simulink model "IntegratedSim2"  (R2018a)
settings: Solver=ode45  StartTime=0.0  StopTime=25  RelTol=1e-7
undefined symbols (not defined in the file or in its folder): Hsys0, qBody0, vp
libraries: vrlib x4, aerolibutil x2, dspmtrx3 x1
settings Model: Creator=henry  LastModifiedBy=henry
settings SolverCC: ConsecutiveZCsStepRelTol=10*128*1  ZeroCrossControl=EnableAll  ZeroCrossAlgorithm=Adaptive

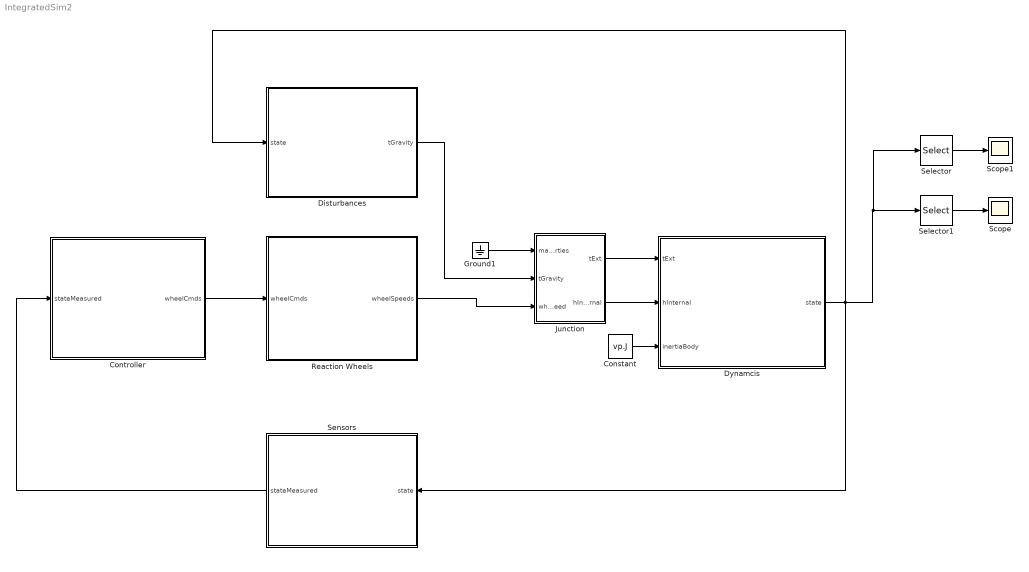
== system IntegratedSim2 ==
  Constant : Constant  Value=vp.J
  Controller : Subsystem
  Disturbances : Subsystem
  Dynamcis : Subsystem
  Ground1 : Ground
  Junction : Subsystem
  Reaction Wheels : Subsystem
  Scope : Scope
  Scope1 : Scope
  Selector : Selector  InputPortWidth=7  IndexOptions=Index vector (dialog)  Indices=[1:4]  OutputSizes=1
  Selector1 : Selector  InputPortWidth=7  IndexOptions=Index vector (dialog)  Indices=[5:7]  OutputSizes=1
  Sensors : Subsystem
  wires:
  Disturbances/1(tGravity) -> Junction/2(tGravity)
  Ground1/1 -> Junction/1(massProperties)
  Junction/1(tExt) -> Dynamcis/1(tExt)
  Controller/1(wheelCmds) -> Reaction Wheels/1(wheelCmds)
  Reaction Wheels/1(wheelSpeeds) -> Junction/3(wheelSpeed)
  Sensors/1(stateMeasured) -> Controller/1(stateMeasured)
  Constant/1 -> Dynamcis/3(inertiaBody)
  Junction/2(hInternal) -> Dynamcis/2(hInternal)
  Dynamcis/1(state) -> Selector/1, Selector1/1, Disturbances/1("state "), Sensors/1(state)
  Selector1/1 -> Scope/1
  Selector/1 -> Scope1/1

== system IntegratedSim2/Controller ==
  stateMeasured : Inport
  wheelCmds : Outport
  wires:
  stateMeasured/1 -> wheelCmds/1

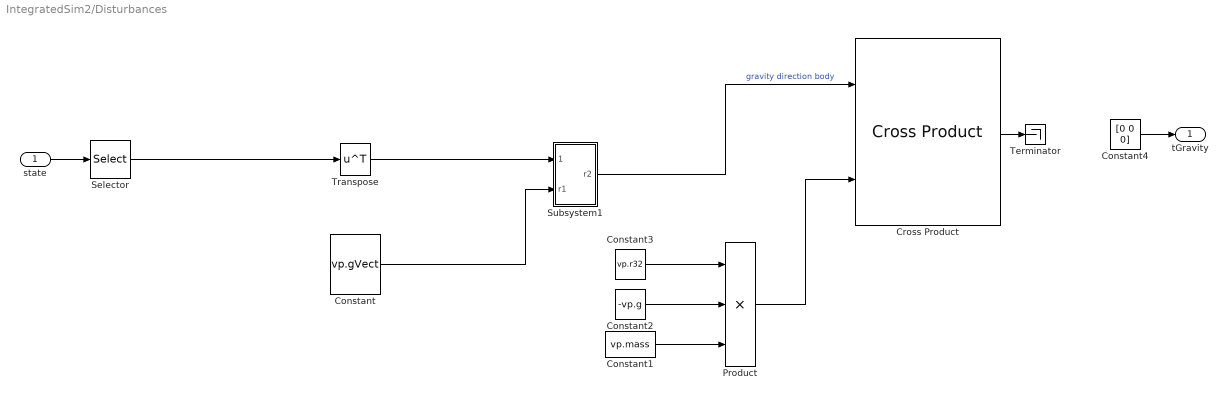
== system IntegratedSim2/Disturbances ==
  "state " : Inport
  Constant : Constant  Value=vp.gVect
  Constant1 : Constant  Value=vp.mass
  Constant2 : Constant  Value=-vp.g
  Constant3 : Constant  Value=vp.r32
  Constant4 : Constant  Value=[0 0 0]
  Cross Product : vrlib/Utilities/Cross Product
      settings: SourceProductBaseCode=VR
  Product : Product  Inputs=3
  Selector : Selector  InputPortWidth=7  IndexOptions=Index vector (dialog)  Indices=[1:4]  OutputSizes=1
  Subsystem1 : Subsystem  mask(Quaternion Transformation){}
      mask help: This blocks transforms the vector r1 from frame a to frame b.
  Terminator : Terminator
  Transpose : Math  Operator=transpose  SaturateOnIntegerOverflow=on
  tGravity : Outport
  wires:
  Constant/1 -> Subsystem1/2(r1)
  Constant1/1 -> Product/3
  Constant2/1 -> Product/2
  Constant3/1 -> Product/1
  Transpose/1 -> Subsystem1/1(qa2b)
  "state "/1 -> Selector/1
  Selector/1 -> Transpose/1
  Product/1 -> Cross Product/2
  Subsystem1/1(r2) -> Cross Product/1  "gravity direction body"
  Constant4/1 -> tGravity/1
  Cross Product/1 -> Terminator/1

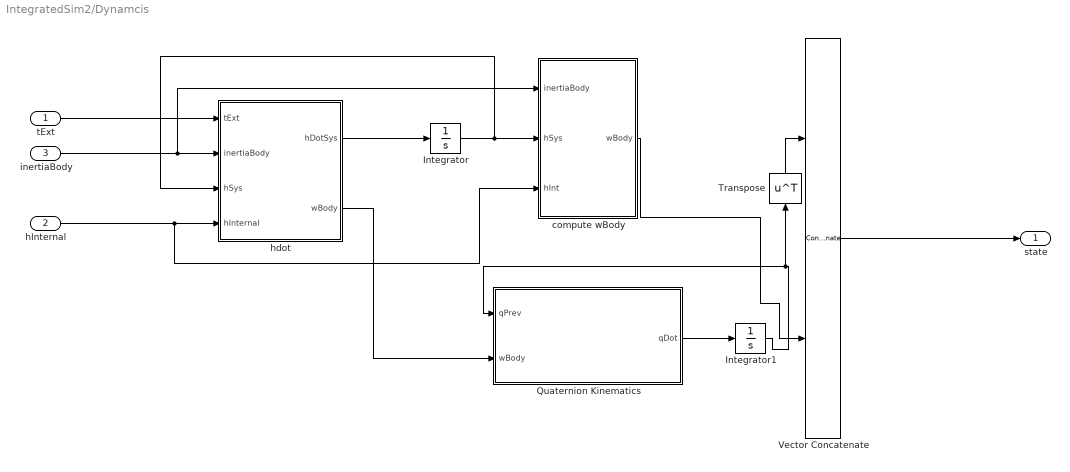
== system IntegratedSim2/Dynamcis ==
  tExt : Inport
  hInternal : Inport  Port=2
  inertiaBody : Inport  Port=3
  Integrator : Integrator  InitialCondition=Hsys0
  Integrator1 : Integrator  InitialCondition=qBody0
  Quaternion Kinematics : Subsystem
  Transpose : Math  Operator=transpose  SaturateOnIntegerOverflow=on
  Vector Concatenate : Concatenate
  compute wBody : Subsystem
  hdot : Subsystem
  state : Outport
  wires:
  hInternal/1 -> compute wBody/3(hInt), hdot/4(hInternal)
  inertiaBody/1 -> compute wBody/1(inertiaBody), hdot/2(inertiaBody)
  tExt/1 -> hdot/1(tExt)
  hdot/1(hDotSys) -> Integrator/1
  Quaternion Kinematics/1(qDot) -> Integrator1/1
  hdot/2(wBody) -> Quaternion Kinematics/2(wBody)
  Integrator/1 -> hdot/3(hSys), compute wBody/2(hSys)
  Integrator1/1 -> Transpose/1, Quaternion Kinematics/1(qPrev)
  Vector Concatenate/1 -> state/1
  compute wBody/1(wBody) -> Vector Concatenate/2
  Transpose/1 -> Vector Concatenate/1

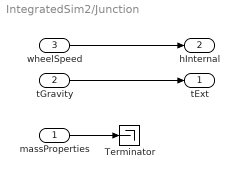
== system IntegratedSim2/Junction ==
  massProperties : Inport
  tGravity : Inport  Port=2
  wheelSpeed : Inport  Port=3
  Terminator : Terminator
  tExt : Outport
  hInternal : Outport  Port=2
  wires:
  wheelSpeed/1 -> hInternal/1
  tGravity/1 -> tExt/1
  massProperties/1 -> Terminator/1

== system IntegratedSim2/Reaction Wheels ==
  wheelCmds : Inport
  Constant : Constant  Value=[0 0 0]
  Terminator : Terminator
  wheelSpeeds : Outport
  wires:
  wheelCmds/1 -> Terminator/1
  Constant/1 -> wheelSpeeds/1

== system IntegratedSim2/Sensors ==
  state : Inport
  stateMeasured : Outport
  wires:
  state/1 -> stateMeasured/1

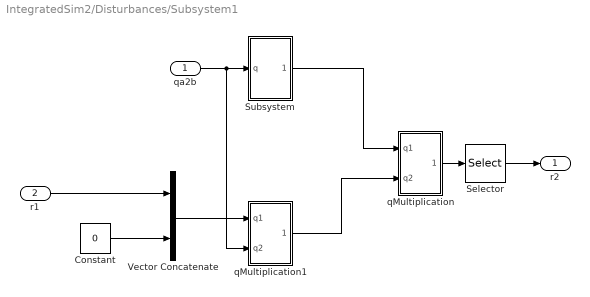
== system IntegratedSim2/Disturbances/Subsystem1 ==
  qa2b : Inport
  r1 : Inport  Port=2
  Constant : Constant  Value=0
  Selector : Selector  InputPortWidth=4  IndexOptions=Index vector (dialog)  Indices=[1:3]  OutputSizes=1
  Subsystem : Subsystem  mask(Quaternion Conjugate){}
      mask help: This block takes the conjugate of the input quaternion
  Vector Concatenate : Concatenate
  qMultiplication : Subsystem  mask(Quaternion Multiplication){}
      mask help: This block performs the quaternion multiplication given two input quaternions.
  qMultiplication1 : Subsystem  mask(Quaternion Multiplication){}
      mask help: This block performs the quaternion multiplication given two input quaternions.
  r2 : Outport
  wires:
  Selector/1 -> r2/1
  qMultiplication/1(q12) -> Selector/1
  qMultiplication1/1(q12) -> qMultiplication/2(q2)
  Vector Concatenate/1 -> qMultiplication1/1(q1)
  Constant/1 -> Vector Concatenate/2
  Subsystem/1(qConj) -> qMultiplication/1(q1)
  qa2b/1 -> Subsystem/1(q), qMultiplication1/2(q2)
  r1/1 -> Vector Concatenate/1

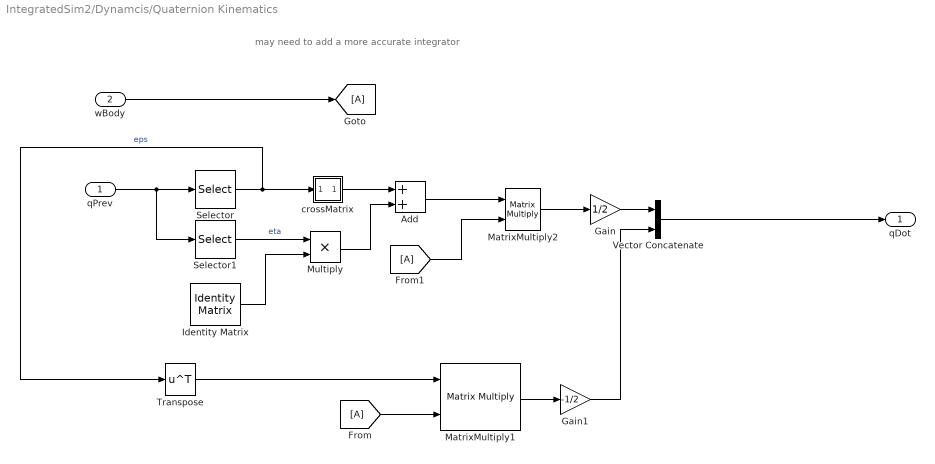
== system IntegratedSim2/Dynamcis/Quaternion Kinematics ==
  note: may need to add a more accurate integrator
  qPrev : Inport
  wBody : Inport  Port=2
  Add : Sum
  Gain : Gain  Gain=1/2
  Gain1 : Gain  Gain=-1/2
  Identity Matrix : dspmtrx3/Identity Matrix  Inherit=off  N=3  Ts=1  dataType=double  isSigned=on  wordLen=16  udDataType=sfix(16)  fracBitsMode=Best precision  numFracBits=15  OutDataTypeStr=double  LastOutDataTypeStr=double
      settings: SourceProductName=DSP System Toolbox
  MatrixMultiply1 : Product  Multiplication=Matrix(*)
  MatrixMultiply2 : Product  Multiplication=Matrix(*)
  Multiply : Product
  Selector : Selector  InputPortWidth=4  IndexOptions=Index vector (dialog)  Indices=[1:3]  OutputSizes=1
  Selector1 : Selector  InputPortWidth=4  IndexOptions=Index vector (dialog)  Indices=4  OutputSizes=1
  Transpose : Math  Operator=transpose  SaturateOnIntegerOverflow=on
  Vector Concatenate : Concatenate
  "crossMatrix " : Subsystem  mask(Cross Matrix){}
      mask help: This block takes in a 3x1 vector and outputs it's corresponding 3x3 cross product matrix
  qDot : Outport
  wires:
  qPrev/1 -> Selector1/1, Selector/1
  Selector/1 -> Transpose/1, "crossMatrix "/1(a)  "eps"
  Selector1/1 -> Multiply/1  "eta"
  Identity Matrix/1 -> Multiply/2
  "crossMatrix "/1(aX) -> Add/1
  Multiply/1 -> Add/2
  Add/1 -> MatrixMultiply2/1
  MatrixMultiply2/1 -> Gain/1
  Gain/1 -> Vector Concatenate/1
  MatrixMultiply1/1 -> Gain1/1
  Gain1/1 -> Vector Concatenate/2
  [A] -> MatrixMultiply1/2
  [A] -> MatrixMultiply2/2
  wBody/1 -> [A]
  Vector Concatenate/1 -> qDot/1
  Transpose/1 -> MatrixMultiply1/1

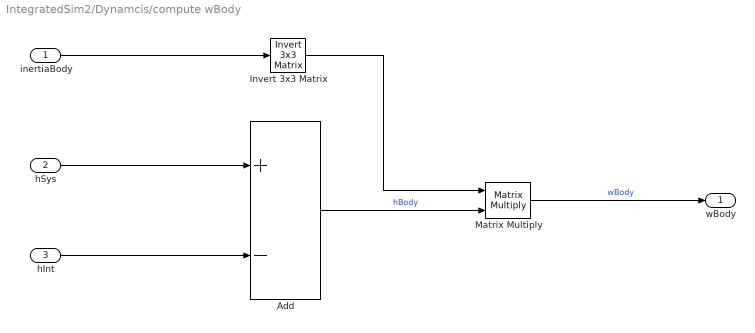
== system IntegratedSim2/Dynamcis/compute wBody ==
  inertiaBody : Inport
  hSys : Inport  Port=2
  hInt : Inport  Port=3
  Add : Sum  Inputs=+-
  Invert 3x3 Matrix : aerolibutil/Invert  3x3 Matrix
  Matrix Multiply : Product  Multiplication=Matrix(*)
  wBody : Outport
  wires:
  inertiaBody/1 -> Invert 3x3 Matrix/1
  hSys/1 -> Add/1
  Matrix Multiply/1 -> wBody/1  "wBody"
  Invert 3x3 Matrix/1 -> Matrix Multiply/1
  hInt/1 -> Add/2
  Add/1 -> Matrix Multiply/2  "hBody"

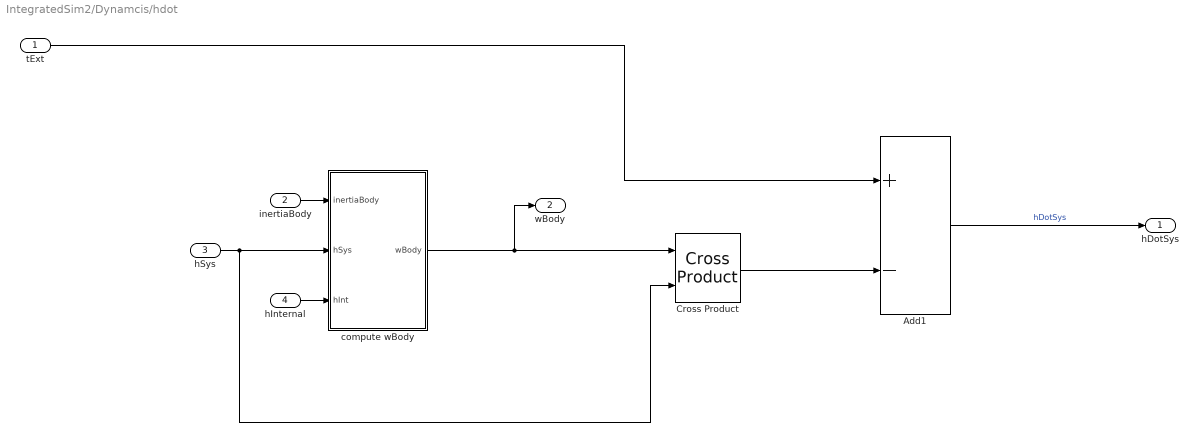
== system IntegratedSim2/Dynamcis/hdot ==
  tExt : Inport
  inertiaBody : Inport  Port=2
  hSys : Inport  Port=3
  hInternal : Inport  Port=4
  Add1 : Sum  Inputs=+-
  Cross Product : vrlib/Utilities/Cross Product
      settings: SourceProductBaseCode=VR
  compute wBody : Subsystem
  hDotSys : Outport
  wBody : Outport  Port=2
  wires:
  Add1/1 -> hDotSys/1  "hDotSys"
  tExt/1 -> Add1/1
  Cross Product/1 -> Add1/2
  inertiaBody/1 -> compute wBody/1(inertiaBody)
  hInternal/1 -> compute wBody/3(hInt)
  compute wBody/1(wBody) -> wBody/1, Cross Product/1
  hSys/1 -> Cross Product/2, compute wBody/2(hSys)

== system IntegratedSim2/Disturbances/Subsystem1/Subsystem ==
  q : Inport
  Gain : Gain  Gain=-1
  Selector : Selector  InputPortWidth=4  IndexOptions=Index vector (dialog)  Indices=[1:3]  OutputSizes=1
  Selector1 : Selector  InputPortWidth=4  IndexOptions=Index vector (dialog)  Indices=4  OutputSizes=1
  Vector Concatenate : Concatenate
  qConj : Outport
  wires:
  Vector Concatenate/1 -> qConj/1
  Gain/1 -> Vector Concatenate/1
  Selector1/1 -> Vector Concatenate/2
  q/1 -> Selector1/1, Selector/1
  Selector/1 -> Gain/1

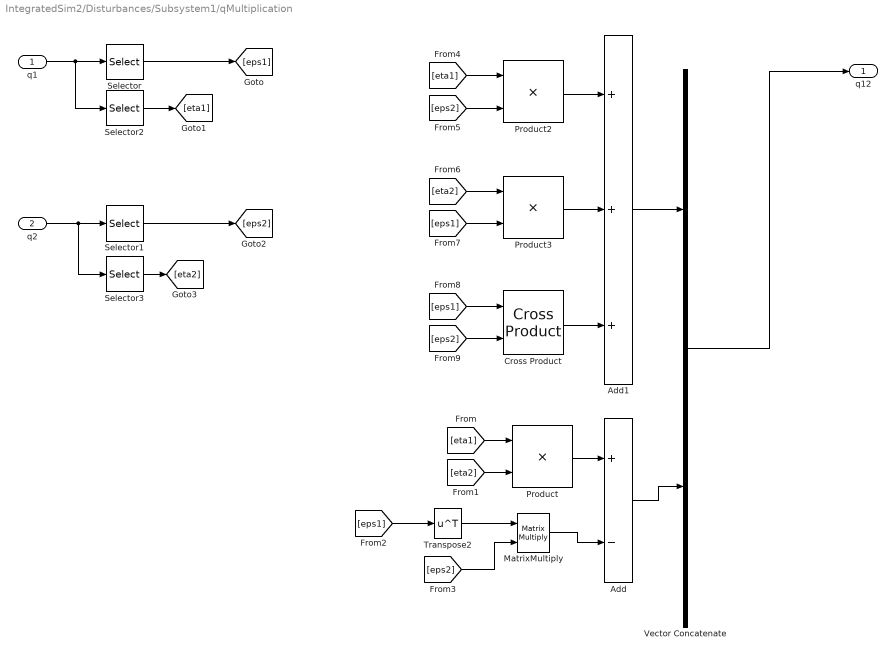
== system IntegratedSim2/Disturbances/Subsystem1/qMultiplication ==
  q1 : Inport
  q2 : Inport  Port=2
  Add : Sum  Inputs=+-
  Add1 : Sum  Inputs=+++
  Cross Product : vrlib/Utilities/Cross Product
      settings: SourceProductBaseCode=VR
  MatrixMultiply : Product  Multiplication=Matrix(*)
  Product : Product
  Product2 : Product
  Product3 : Product
  Selector : Selector  InputPortWidth=4  IndexOptions=Index vector (dialog)  Indices=[1:3]  OutputSizes=1
  Selector1 : Selector  InputPortWidth=4  IndexOptions=Index vector (dialog)  Indices=[1:3]  OutputSizes=1
  Selector2 : Selector  InputPortWidth=4  IndexOptions=Index vector (dialog)  Indices=4  OutputSizes=1
  Selector3 : Selector  InputPortWidth=4  IndexOptions=Index vector (dialog)  Indices=4  OutputSizes=1
  Transpose2 : Math  Operator=transpose  SaturateOnIntegerOverflow=on
  Vector Concatenate : Concatenate
  q12 : Outport
  wires:
  Selector3/1 -> [eta2]
  Product2/1 -> Add1/1
  Product/1 -> Add/1
  [eta1] -> Product2/1
  [eta2] -> Product/2
  Product3/1 -> Add1/2
  q1/1 -> Selector2/1, Selector/1
  Transpose2/1 -> MatrixMultiply/1
  Selector2/1 -> [eta1]
  Selector1/1 -> [eps2]
  Cross Product/1 -> Add1/3
  [eps1] -> Transpose2/1
  q2/1 -> Selector3/1, Selector1/1
  [eta2] -> Product3/1
  [eta1] -> Product/1
  Vector Concatenate/1 -> q12/1
  [eps2] -> Product2/2
  [eps1] -> Product3/2
  Selector/1 -> [eps1]
  [eps2] -> Cross Product/2
  MatrixMultiply/1 -> Add/2
  [eps1] -> Cross Product/1
  [eps2] -> MatrixMultiply/2
  Add1/1 -> Vector Concatenate/1
  Add/1 -> Vector Concatenate/2

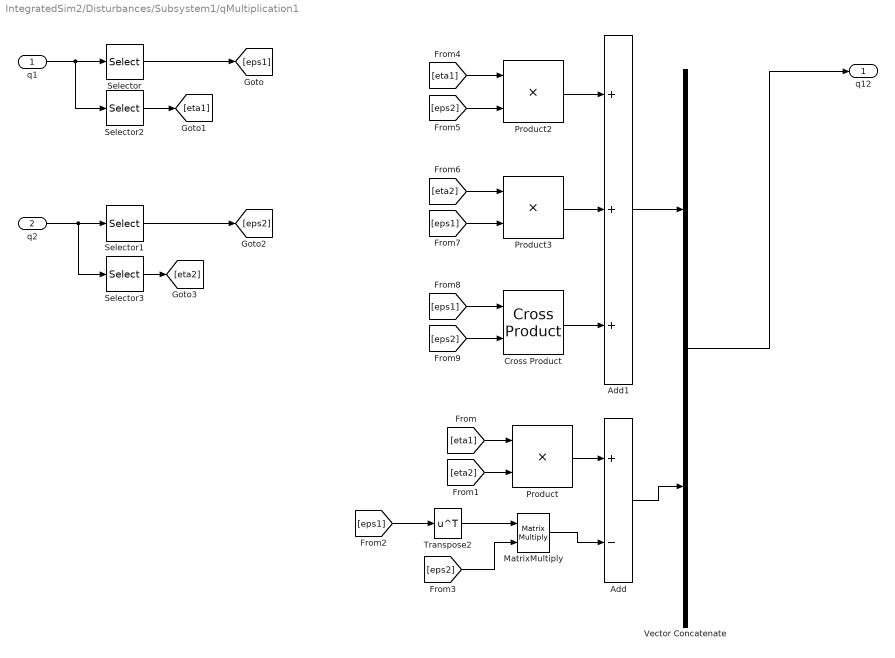
== system IntegratedSim2/Disturbances/Subsystem1/qMultiplication1 ==
  q1 : Inport
  q2 : Inport  Port=2
  Add : Sum  Inputs=+-
  Add1 : Sum  Inputs=+++
  Cross Product : vrlib/Utilities/Cross Product
      settings: SourceProductBaseCode=VR
  MatrixMultiply : Product  Multiplication=Matrix(*)
  Product : Product
  Product2 : Product
  Product3 : Product
  Selector : Selector  InputPortWidth=4  IndexOptions=Index vector (dialog)  Indices=[1:3]  OutputSizes=1
  Selector1 : Selector  InputPortWidth=4  IndexOptions=Index vector (dialog)  Indices=[1:3]  OutputSizes=1
  Selector2 : Selector  InputPortWidth=4  IndexOptions=Index vector (dialog)  Indices=4  OutputSizes=1
  Selector3 : Selector  InputPortWidth=4  IndexOptions=Index vector (dialog)  Indices=4  OutputSizes=1
  Transpose2 : Math  Operator=transpose  SaturateOnIntegerOverflow=on
  Vector Concatenate : Concatenate
  q12 : Outport
  wires:
  Add/1 -> Vector Concatenate/2
  Add1/1 -> Vector Concatenate/1
  [eps2] -> MatrixMultiply/2
  [eps1] -> Cross Product/1
  MatrixMultiply/1 -> Add/2
  [eps2] -> Cross Product/2
  Selector/1 -> [eps1]
  [eps1] -> Product3/2
  [eps2] -> Product2/2
  Vector Concatenate/1 -> q12/1
  [eta1] -> Product/1
  [eta2] -> Product3/1
  q2/1 -> Selector1/1, Selector3/1
  [eps1] -> Transpose2/1
  Cross Product/1 -> Add1/3
  Selector1/1 -> [eps2]
  Selector2/1 -> [eta1]
  Transpose2/1 -> MatrixMultiply/1
  q1/1 -> Selector/1, Selector2/1
  Product3/1 -> Add1/2
  [eta2] -> Product/2
  [eta1] -> Product2/1
  Product/1 -> Add/1
  Product2/1 -> Add1/1
  Selector3/1 -> [eta2]

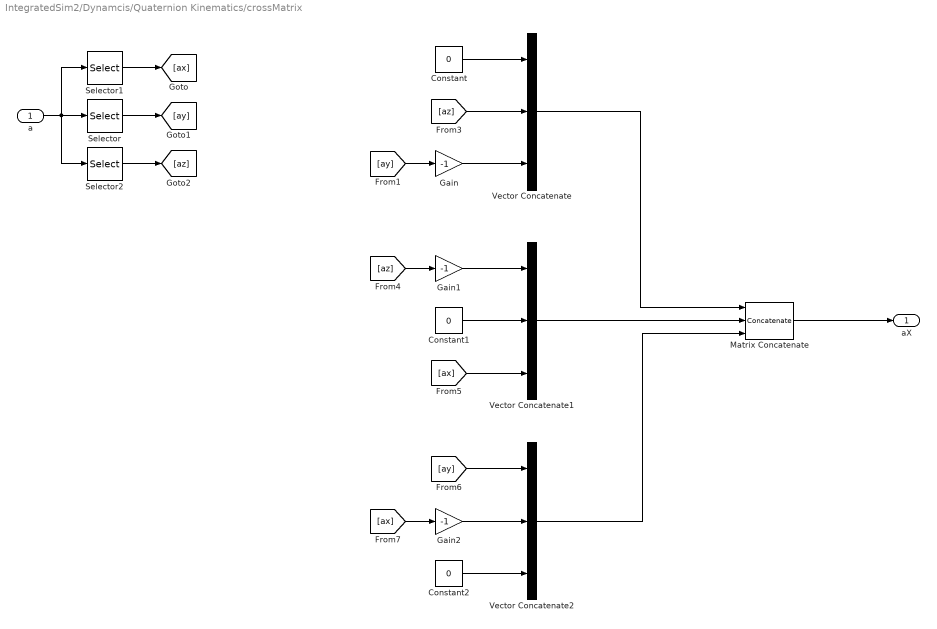
== system IntegratedSim2/Dynamcis/Quaternion Kinematics/crossMatrix  ==
  a : Inport
  Constant : Constant  Value=0
  Constant1 : Constant  Value=0
  Constant2 : Constant  Value=0
  Gain : Gain  Gain=-1
  Gain1 : Gain  Gain=-1
  Gain2 : Gain  Gain=-1
  Matrix Concatenate : Concatenate  NumInputs=3  Mode=Multidimensional array  ConcatenateDimension=2
  Selector : Selector  InputPortWidth=3  IndexOptions=Index vector (dialog)  Indices=2  OutputSizes=1
  Selector1 : Selector  InputPortWidth=3  IndexOptions=Index vector (dialog)  Indices=1  OutputSizes=1
  Selector2 : Selector  InputPortWidth=3  IndexOptions=Index vector (dialog)  Indices=3  OutputSizes=1
  Vector Concatenate : Concatenate  NumInputs=3
  Vector Concatenate1 : Concatenate  NumInputs=3
  Vector Concatenate2 : Concatenate  NumInputs=3
  aX : Outport
  wires:
  [ay] -> Gain/1
  [az] -> Gain1/1
  Gain2/1 -> Vector Concatenate2/2
  Constant1/1 -> Vector Concatenate1/2
  [ax] -> Vector Concatenate1/3
  [ay] -> Vector Concatenate2/1
  Vector Concatenate1/1 -> Matrix Concatenate/2
  Matrix Concatenate/1 -> aX/1
  Constant2/1 -> Vector Concatenate2/3
  [ax] -> Gain2/1
  Vector Concatenate2/1 -> Matrix Concatenate/3
  Gain/1 -> Vector Concatenate/3
  Vector Concatenate/1 -> Matrix Concatenate/1
  Selector1/1 -> [ax]
  Selector2/1 -> [az]
  [az] -> Vector Concatenate/2
  Gain1/1 -> Vector Concatenate1/1
  Constant/1 -> Vector Concatenate/1
  a/1 -> Selector/1, Selector1/1, Selector2/1
  Selector/1 -> [ay]

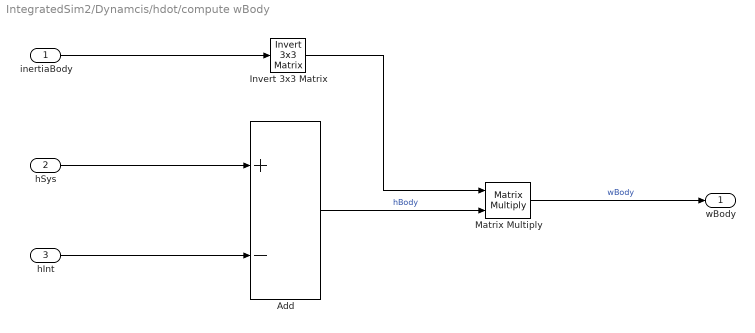
== system IntegratedSim2/Dynamcis/hdot/compute wBody ==
  inertiaBody : Inport
  hSys : Inport  Port=2
  hInt : Inport  Port=3
  Add : Sum  Inputs=+-
  Invert 3x3 Matrix : aerolibutil/Invert  3x3 Matrix
  Matrix Multiply : Product  Multiplication=Matrix(*)
  wBody : Outport
  wires:
  inertiaBody/1 -> Invert 3x3 Matrix/1
  hSys/1 -> Add/1
  Matrix Multiply/1 -> wBody/1  "wBody"
  Invert 3x3 Matrix/1 -> Matrix Multiply/1
  hInt/1 -> Add/2
  Add/1 -> Matrix Multiply/2  "hBody"
